simulink model "work1"  (R2022b)
settings: Solver=VariableStepAuto  StartTime=0.0  StopTime=2000  RelTol=1e-3
settings Model: Creator=Administrator  LastModifiedBy=Administrator

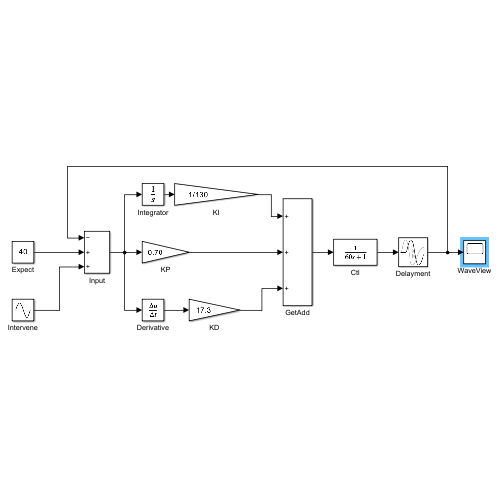
[thumbnail: Simulink's stored preview of the top-level diagram]
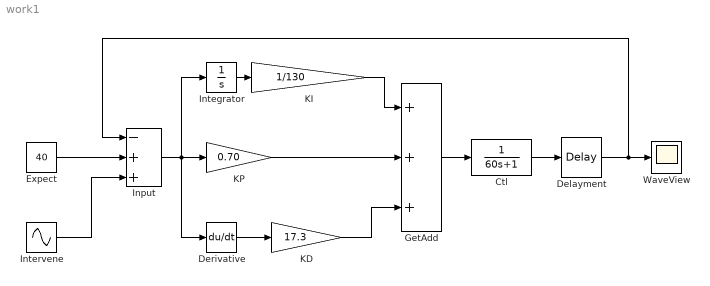
== system work1 ==
  Ctl : TransferFcn  Denominator=[60 1]
  Delayment : TransportDelay  DelayTime=80
  Derivative : Derivative
  Expect : Constant  Value=40
  GetAdd : Sum  Inputs=+++
  Input : Sum  Inputs=-++
  Integrator : Integrator
  Intervene : Sin  Amplitude=0.05  Frequency=500  SampleTime=0
  KD : Gain  Gain=17.3
  KI : Gain  Gain=1/130
  KP : Gain  Gain=0.70
  WaveView : Scope
  wires:
  Expect/1 -> Input/2
  Input/1 -> Derivative/1, Integrator/1, KP/1
  Integrator/1 -> KI/1
  Ctl/1 -> Delayment/1
  Delayment/1 -> Input/1, WaveView/1
  Derivative/1 -> KD/1
  GetAdd/1 -> Ctl/1
  Intervene/1 -> Input/3
  KP/1 -> GetAdd/2
  KI/1 -> GetAdd/1
  KD/1 -> GetAdd/3
